simulink model "TPN"  (R2024b)
settings: Solver=ode45  StartTime=0.0  StopTime=20.0  MaxStep=1E-3  RelTol=1e-3
libraries: slpidlib x1
settings Model: Creator=leslie  LastModifiedBy=leslie
settings DataIOCC: ReturnWorkspaceOutputs=off  TimeSaveName=t  OutputSaveName=y
settings DebuggingCC: AlgebraicLoopMsg=none  ArtificialAlgebraicLoopMsg=none  MaxConsecutiveZCsMsg=none  OperatingPointInterfaceChecksumMismatchMsg=none

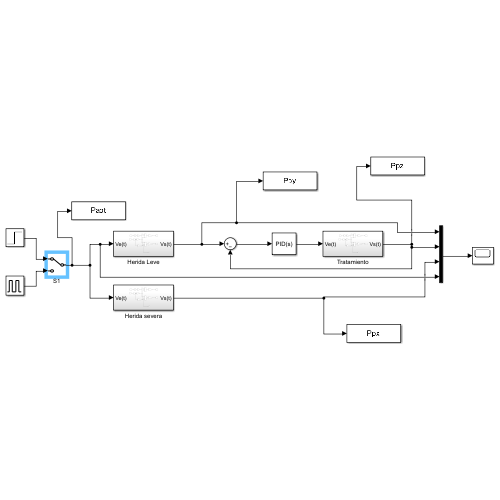
[thumbnail: Simulink's stored preview of the top-level diagram]
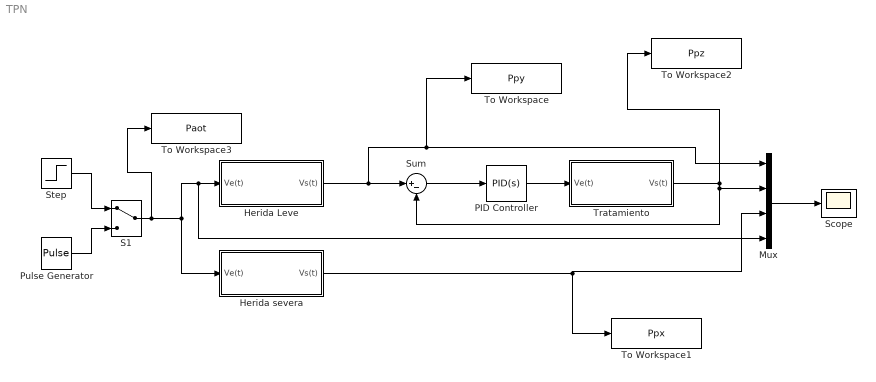
== system TPN ==
  Herida Leve : Subsystem
  Herida severa : Subsystem
  Mux : Mux
  PID Controller : slpidlib/PID Controller  Controller=PID  Form=Parallel  TimeDomain=Continuous-time  UseExternalTs=off  SampleTime=-1  IntegratorMethod=Forward Euler  FilterMethod=Forward Euler  ControllerParametersSource=internal  P=721.192634314108  I=271.444293310424  UseKiTs=off  D=425.738397034128  UseExternalDerivativeSource=off  N=7373.08371639744  UseFilter=on  TunerSelectOption=Transfer Function Based (PID Tuner App)  InitialConditionSource=internal  InitialConditionForIntegrator=0  InitialConditionForFilter=0  DifferentiatorICPrevScaledInput=0  ExternalReset=none  TrackingMode=off  Kt=1  LimitOutput=off  SatLimitsSource=internal  UpperSaturationLimit=inf  LowerSaturationLimit=-inf  LinearizeAsGain=on  AntiWindupMode=none  Kb=1  LimitIntegrator=off  UpperIntegratorSaturationLimit=inf  LowerIntegratorSaturationLimit=-inf  POutMin=[]  POutMax=[]  IOutMin=[]  IOutMax=[]  DOutMin=[]  DOutMax=[]  NOutMin=[]  NOutMax=[]  SumOutMin=[]  SumOutMax=[]  SaturationOutMin=[]  SaturationOutMax=[]  PParamMin=[]  PParamMax=[]  IParamMin=[]  IParamMax=[]  DParamMin=[]  DParamMax=[]  NParamMin=[]  NParamMax=[]  KbParamMin=[]  KbParamMax=[]  KtParamMin=[]  KtParamMax=[]  KbOutMin=[]  KbOutMax=[]  KtOutMin=[]  KtOutMax=[]  IntegratorOutMin=[]  IntegratorOutMax=[]  FilterOutMin=[]  FilterOutMax=[]  SumI1OutMin=[]  SumI1OutMax=[]  SumI2OutMin=[]  SumI2OutMax=[]  SumI3OutMin=[]  SumI3OutMax=[]  SumI4OutMin=[]  SumI4OutMax=[]  SumDOutMin=[]  SumDOutMax=[]  DifferentiatorOutMin=[]  DifferentiatorOutMax=[]  FilterDiffOutCoefMin=[]  FilterDiffOutCoefMax=[]  ReciprocalOutMin=[]  ReciprocalOutMax=[]  SumDenOutMin=[]  SumDenOutMax=[]  SumNumOutMin=[]  SumNumOutMax=[]  DivideOutMin=[]  DivideOutMax=[]  UdiffTsProdOutMin=[]  UdiffTsProdOutMax=[]  NTsProdOutMin=[]  NTsProdOutMax=[]  UintegralTsProdOutMin=[]  UintegralTsProdOutMax=[]  UngainTsProdOutMin=[]  UngainTsProdOutMax=[]  ClampingZeroOutDataTypeStr=Inherit: Inherit via back propagation  ClampingZeroOutMin=[]  ClampingZeroOutMax=[]  FilterDenConstantOutDataTypeStr=Inherit: Inherit via back propagation  FilterDenConstantOutMin=[]  FilterDenConstantOutMax=[]  PCopyOutDataTypeStr=Inherit: Inherit via back propagation  PCopyOutMin=[]  PCopyOutMax=[]  NCopyOutDataTypeStr=Inherit: Inherit via back propagation  NCopyOutMin=[]  NCopyOutMax=[]  IntegratorContinuousStateAttributes=''  IntegratorStateMustResolveToSignalObject=off  IntegratorRTWStateStorageClass=Auto  FilterContinuousStateAttributes=''  FilterStateMustResolveToSignalObject=off  FilterRTWStateStorageClass=Auto  ParallelPVariant=InternalParameters  IdealPVariant=Disabled  IVariant=InternalParameters  DVariant=InternalParameters  IntegratorVariant=Continuous  SatVariant=Disabled  AWVariant=Passthrough  PCopyVariant=Disabled  TRVariant=Disabled  FdbkBlocksVariant=Forward  IdealPFdbkVariant=Disabled  SatFdbkVariant=Disabled  DerivativeFilterVariant=ContFilter  NVariant=InternalParameters  NCopyVariant=Disabled  FilterICVariant=InternalICsFilter  IntegratorICVariant=InternalICs  ExternalResetVariant=Disabled  TRSumVariant=Passthrough  SumFdbkVariant=Disabled  SumVariant=Sum_PID  TsampFilterVariant=InternalTs  TsampNgainVariant=Passthrough  TsampIntegralVariant=Disabled_SignalSpec  ExternalSaturationOutDataTypeStr=Inherit: Same as second input  DerivativeSourceVariant=ErrorSignal  PreIntVariant=InternalPreInt
  Pulse Generator : DiscretePulseGenerator  PulseType=Time based  Period=20  PulseWidth=10
  S1 : ManualSwitch
  Scope : Scope
  Step : Step  Time=0  SampleTime=0
  Sum : Sum  Inputs=|+-
  To Workspace : ToWorkspace  VariableName=Ppy  SaveFormat=Timeseries  SampleTime=-1
  To Workspace1 : ToWorkspace  VariableName=Ppx  SaveFormat=Timeseries  SampleTime=-1
  To Workspace2 : ToWorkspace  VariableName=Ppz  SaveFormat=Timeseries  SampleTime=-1
  To Workspace3 : ToWorkspace  VariableName=Paot  SaveFormat=Timeseries  SampleTime=-1
  Tratamiento : Subsystem
  wires:
  Step/1 -> S1/1
  Pulse Generator/1 -> S1/2
  PID Controller/1 -> Tratamiento/1(Ve(t))
  Sum/1 -> PID Controller/1
  Herida Leve/1(Vs(t)) -> To Workspace/1, Mux/1, Sum/1
  S1/1 -> To Workspace3/1, Herida severa/1(Ve(t)), Mux/4, Herida Leve/1(Ve(t))
  Mux/1 -> Scope/1
  Herida severa/1(Vs(t)) -> To Workspace1/1, Mux/3
  Tratamiento/1(Vs(t)) -> To Workspace2/1, Sum/2, Mux/2

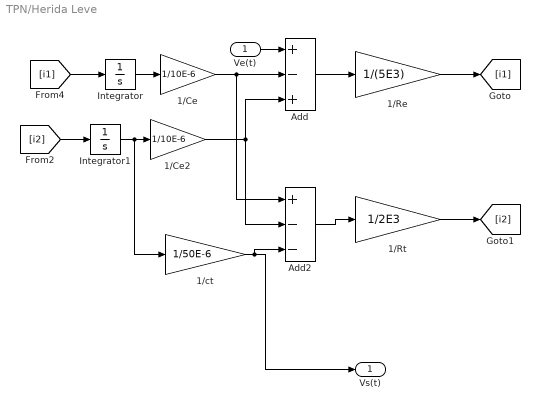
== system TPN/Herida Leve ==
  Ve(t) : Inport
  1/Ce : Gain  Gain=1/10E-6
  1/Ce2 : Gain  Gain=1/10E-6
  1/Re : Gain  Gain=1/(5E3)
  1/Rt : Gain  Gain=1/2E3
  1/ct : Gain  Gain=1/50E-6
  Add : Sum  Inputs=+-+
  Add2 : Sum  Inputs=+--
  Integrator : Integrator
  Integrator1 : Integrator
  Vs(t) : Outport
  wires:
  Add/1 -> 1/Re/1
  1/Ce/1 -> Add2/1, Add/2
  Ve(t)/1 -> Add/1
  1/Ce2/1 -> Add2/2, Add/3
  1/ct/1 -> Add2/3, Vs(t)/1
  1/Rt/1 -> [i2]
  1/Re/1 -> [i1]
  Add2/1 -> 1/Rt/1
  Integrator/1 -> 1/Ce/1
  [i1] -> Integrator/1
  Integrator1/1 -> 1/ct/1, 1/Ce2/1
  [i2] -> Integrator1/1

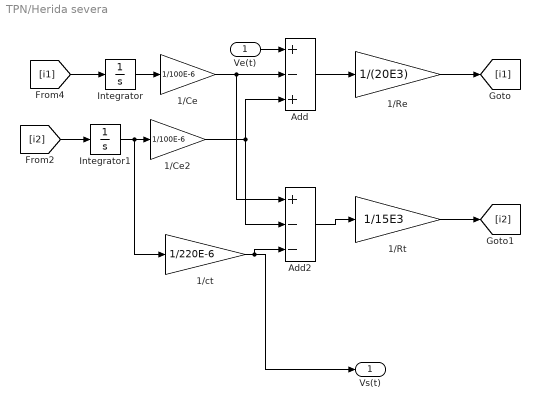
== system TPN/Herida severa ==
  Ve(t) : Inport
  1/Ce : Gain  Gain=1/100E-6
  1/Ce2 : Gain  Gain=1/100E-6
  1/Re : Gain  Gain=1/(20E3)
  1/Rt : Gain  Gain=1/15E3
  1/ct : Gain  Gain=1/220E-6
  Add : Sum  Inputs=+-+
  Add2 : Sum  Inputs=+--
  Integrator : Integrator
  Integrator1 : Integrator
  Vs(t) : Outport
  wires:
  Integrator/1 -> 1/Ce/1
  [i1] -> Integrator/1
  [i2] -> Integrator1/1
  Add2/1 -> 1/Rt/1
  1/ct/1 -> Add2/3, Vs(t)/1
  1/Ce2/1 -> Add2/2, Add/3
  Integrator1/1 -> 1/ct/1, 1/Ce2/1
  1/Re/1 -> [i1]
  1/Ce/1 -> Add2/1, Add/2
  Ve(t)/1 -> Add/1
  Add/1 -> 1/Re/1
  1/Rt/1 -> [i2]

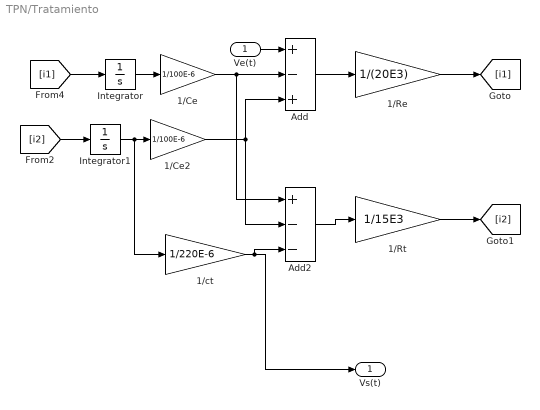
== system TPN/Tratamiento ==
  Ve(t) : Inport
  1/Ce : Gain  Gain=1/100E-6
  1/Ce2 : Gain  Gain=1/100E-6
  1/Re : Gain  Gain=1/(20E3)
  1/Rt : Gain  Gain=1/15E3
  1/ct : Gain  Gain=1/220E-6
  Add : Sum  Inputs=+-+
  Add2 : Sum  Inputs=+--
  Integrator : Integrator
  Integrator1 : Integrator
  Vs(t) : Outport
  wires:
  1/Ce2/1 -> Add2/2, Add/3
  1/ct/1 -> Add2/3, Vs(t)/1
  Add2/1 -> 1/Rt/1
  [i2] -> Integrator1/1
  [i1] -> Integrator/1
  Integrator/1 -> 1/Ce/1
  Ve(t)/1 -> Add/1
  1/Ce/1 -> Add2/1, Add/2
  1/Re/1 -> [i1]
  Integrator1/1 -> 1/ct/1, 1/Ce2/1
  1/Rt/1 -> [i2]
  Add/1 -> 1/Re/1
